simulink model "Estabilidad"  (R2023b)
settings: Solver=VariableStepAuto  StartTime=0.0  StopTime=10.0  RelTol=1e-3
settings Model: Creator=diavl  LastModifiedBy=diavl

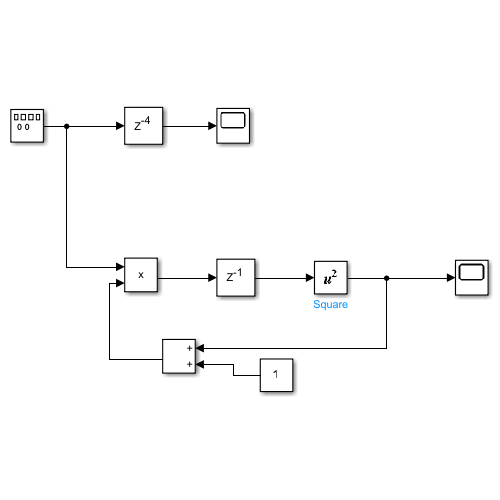
[thumbnail: Simulink's stored preview of the top-level diagram]
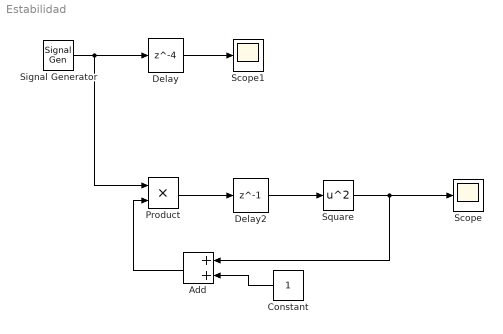
== system Estabilidad ==
  Add : Sum
  Constant : Constant
  Delay : Delay  DelayLength=4  InitialCondition=0
  Delay2 : Delay  DelayLength=1  InitialCondition=0
  Product : Product
  Scope : Scope
  Scope1 : Scope
  Signal Generator : SignalGenerator  WaveForm=random  Amplitude=2  Frequency=2
  Square : Math  Operator=square
  wires:
  Delay/1 -> Scope1/1
  Product/1 -> Delay2/1
  Signal Generator/1 -> Product/1, Delay/1
  Add/1 -> Product/2
  Constant/1 -> Add/2
  Delay2/1 -> Square/1
  Square/1 -> Add/1, Scope/1
